simulink model "TST_CoTS_ThermDem"  (R2016b)
settings: Solver=FixedStepDiscrete  StartTime=0.0  StopTime=simTime  FixedStep=sampleTime  RelTol=1e-3
values from neighbouring files (symbols this model uses):
  testCase = 1    [initTST_CoTS_ThermDem_001.m]
libraries: simulink x4, UnitTest_Lib x2
settings Model: Creator=xinchangran  LastModifiedBy=xinchangran
settings DebuggingCC: SignalRangeChecking=error

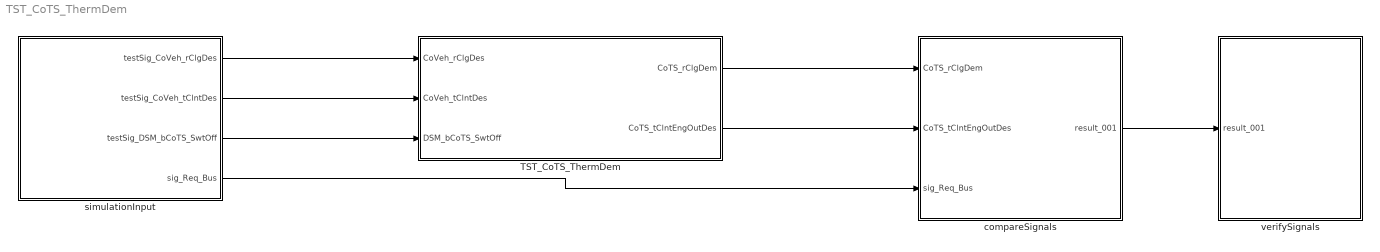
== system TST_CoTS_ThermDem ==
  TST_CoTS_ThermDem : Subsystem
  compareSignals : Subsystem
  simulationInput : Subsystem
  verifySignals : Subsystem
  wires:
  simulationInput/1(testSig_CoVeh_rClgDes) -> TST_CoTS_ThermDem/1(CoVeh_rClgDes)
  simulationInput/2(testSig_CoVeh_tClntDes) -> TST_CoTS_ThermDem/2(CoVeh_tClntDes)
  simulationInput/3(testSig_DSM_bCoTS_SwtOff) -> TST_CoTS_ThermDem/3(DSM_bCoTS_SwtOff)
  TST_CoTS_ThermDem/1(CoTS_rClgDem) -> compareSignals/1(CoTS_rClgDem)
  TST_CoTS_ThermDem/2(CoTS_tClntEngOutDes) -> compareSignals/2(CoTS_tClntEngOutDes)
  simulationInput/4(sig_Req_Bus) -> compareSignals/3(sig_Req_Bus)
  compareSignals/1(result_001) -> verifySignals/1(result_001)

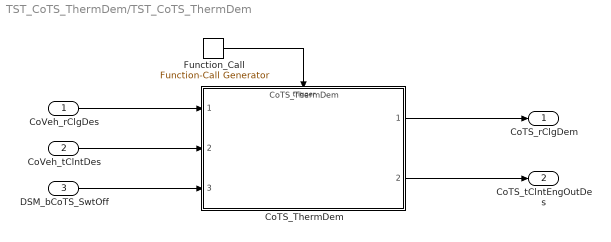
== system TST_CoTS_ThermDem/TST_CoTS_ThermDem ==
  CoVeh_rClgDes : Inport
  CoVeh_tClntDes : Inport  Port=2
  DSM_bCoTS_SwtOff : Inport  Port=3
  CoTS_ThermDem : ModelReference  ModelNameDialog=CoTS_ThermDem  SimulationMode=Normal  ModelReferenceVersion=1.28  TriggerPortName=function  TriggerPortTriggerType=function-call  TriggerPortStatesWhenEnabling=held
  Function_Call : simulink/Ports & Subsystems/Function-Call Generator  sample_time=sampleTime  numberOfIterations=1
  CoTS_rClgDem : Outport
  CoTS_tClntEngOutDes : Outport  Port=2
  wires:
  Function_Call/1 -> CoTS_ThermDem/Trigger
  CoVeh_rClgDes/1 -> CoTS_ThermDem/1
  CoVeh_tClntDes/1 -> CoTS_ThermDem/2
  DSM_bCoTS_SwtOff/1 -> CoTS_ThermDem/3
  CoTS_ThermDem/1 -> CoTS_rClgDem/1
  CoTS_ThermDem/2 -> CoTS_tClntEngOutDes/1

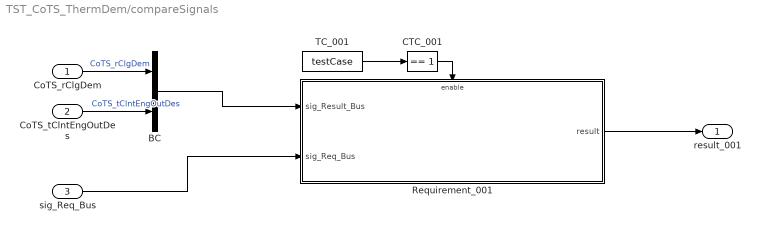
== system TST_CoTS_ThermDem/compareSignals ==
  CoTS_rClgDem : Inport
  CoTS_tClntEngOutDes : Inport  Port=2
  sig_Req_Bus : Inport  Port=3
  BC : BusCreator  Inputs=2
  CTC_001 : simulink/Logic and Bit Operations/Compare To Constant  relop===  const=1  OutDataTypeStr=boolean
  Requirement_001 : Subsystem
  TC_001 : Constant  Value=testCase
  result_001 : Outport
  wires:
  CoTS_rClgDem/1 -> BC/1  "CoTS_rClgDem"
  CoTS_tClntEngOutDes/1 -> BC/2  "CoTS_tClntEngOutDes"
  TC_001/1 -> CTC_001/1
  CTC_001/1 -> Requirement_001/Enable
  sig_Req_Bus/1 -> Requirement_001/2(sig_Req_Bus)
  BC/1 -> Requirement_001/1(sig_Result_Bus)
  Requirement_001/1(result) -> result_001/1

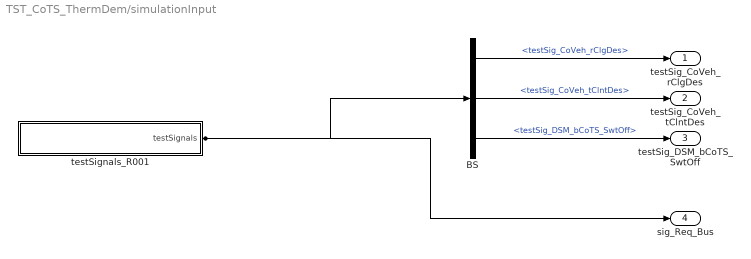
== system TST_CoTS_ThermDem/simulationInput ==
  BS : BusSelector  OutputSignals=testSig_CoVeh_rClgDes,testSig_CoVeh_tClntDes,testSig_DSM_bCoTS_SwtOff
  testSignals_R001 : Subsystem
  testSig_CoVeh_rClgDes : Outport
  testSig_CoVeh_tClntDes : Outport  Port=2
  testSig_DSM_bCoTS_SwtOff : Outport  Port=3
  sig_Req_Bus : Outport  Port=4
  wires:
  BS/1 -> testSig_CoVeh_rClgDes/1  "<testSig_CoVeh_rClgDes>"
  BS/2 -> testSig_CoVeh_tClntDes/1  "<testSig_CoVeh_tClntDes>"
  BS/3 -> testSig_DSM_bCoTS_SwtOff/1  "<testSig_DSM_bCoTS_SwtOff>"
  testSignals_R001/1(testSignals) -> BS/1, sig_Req_Bus/1

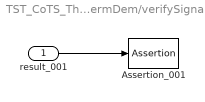
== system TST_CoTS_ThermDem/verifySignals ==
  result_001 : Inport
  Assertion_001 : Assertion  Enabled=off
  wires:
  result_001/1 -> Assertion_001/1

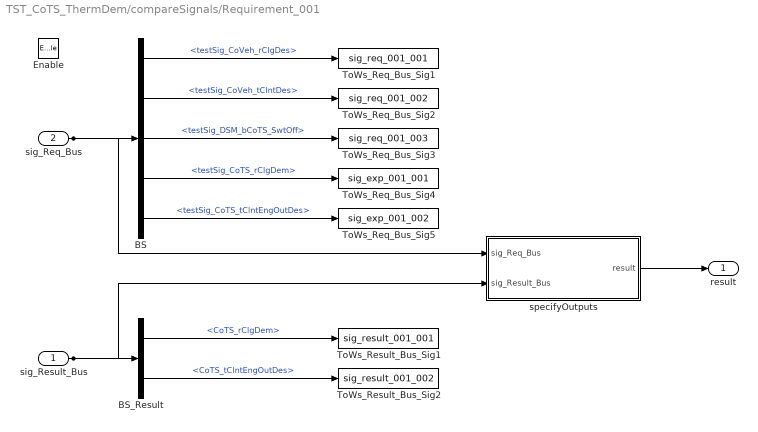
== system TST_CoTS_ThermDem/compareSignals/Requirement_001 ==
  sig_Result_Bus : Inport
  sig_Req_Bus : Inport  Port=2
  Enable : EnablePort
  BS : BusSelector  OutputSignals=testSig_CoVeh_rClgDes,testSig_CoVeh_tClntDes,testSig_DSM_bCoTS_SwtOff,testSig_CoTS_rClgDem,testSig_CoTS_tClntEngOutDes
  BS_Result : BusSelector  OutputSignals=CoTS_rClgDem,CoTS_tClntEngOutDes
  ToWs_Req_Bus_Sig1 : ToWorkspace  VariableName=sig_req_001_001  SaveFormat=Structure With Time
  ToWs_Req_Bus_Sig2 : ToWorkspace  VariableName=sig_req_001_002  SaveFormat=Structure With Time
  ToWs_Req_Bus_Sig3 : ToWorkspace  VariableName=sig_req_001_003  SaveFormat=Structure With Time
  ToWs_Req_Bus_Sig4 : ToWorkspace  VariableName=sig_exp_001_001  SaveFormat=Structure With Time
  ToWs_Req_Bus_Sig5 : ToWorkspace  VariableName=sig_exp_001_002  SaveFormat=Structure With Time
  ToWs_Result_Bus_Sig1 : ToWorkspace  VariableName=sig_result_001_001  SaveFormat=Structure With Time
  ToWs_Result_Bus_Sig2 : ToWorkspace  VariableName=sig_result_001_002  SaveFormat=Structure With Time
  specifyOutputs : Subsystem
  result : Outport
  wires:
  sig_Req_Bus/1 -> BS/1, specifyOutputs/1(sig_Req_Bus)
  BS/1 -> ToWs_Req_Bus_Sig1/1  "<testSig_CoVeh_rClgDes>"
  BS/2 -> ToWs_Req_Bus_Sig2/1  "<testSig_CoVeh_tClntDes>"
  BS/3 -> ToWs_Req_Bus_Sig3/1  "<testSig_DSM_bCoTS_SwtOff>"
  BS/4 -> ToWs_Req_Bus_Sig4/1  "<testSig_CoTS_rClgDem>"
  BS/5 -> ToWs_Req_Bus_Sig5/1  "<testSig_CoTS_tClntEngOutDes>"
  sig_Result_Bus/1 -> BS_Result/1, specifyOutputs/2(sig_Result_Bus)
  BS_Result/1 -> ToWs_Result_Bus_Sig1/1  "<CoTS_rClgDem>"
  BS_Result/2 -> ToWs_Result_Bus_Sig2/1  "<CoTS_tClntEngOutDes>"
  specifyOutputs/1(result) -> result/1

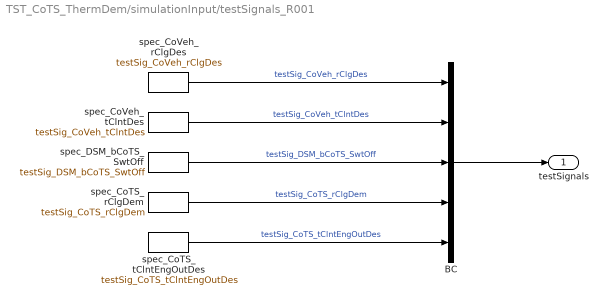
== system TST_CoTS_ThermDem/simulationInput/testSignals_R001 ==
  BC : BusCreator  Inputs=5
  spec_CoTS_rClgDem : FromWorkspace  VariableName=testSig_CoTS_rClgDem  Interpolate=off  OutputAfterFinalValue=Holding final value
  spec_CoTS_tClntEngOutDes : FromWorkspace  VariableName=testSig_CoTS_tClntEngOutDes  Interpolate=off  OutputAfterFinalValue=Holding final value
  spec_CoVeh_rClgDes : FromWorkspace  VariableName=testSig_CoVeh_rClgDes  Interpolate=off  OutputAfterFinalValue=Holding final value
  spec_CoVeh_tClntDes : FromWorkspace  VariableName=testSig_CoVeh_tClntDes  Interpolate=off  OutputAfterFinalValue=Holding final value
  spec_DSM_bCoTS_SwtOff : FromWorkspace  VariableName=testSig_DSM_bCoTS_SwtOff  Interpolate=off  OutputAfterFinalValue=Holding final value
  testSignals : Outport
  wires:
  BC/1 -> testSignals/1
  spec_CoVeh_rClgDes/1 -> BC/1  "testSig_CoVeh_rClgDes"
  spec_CoVeh_tClntDes/1 -> BC/2  "testSig_CoVeh_tClntDes"
  spec_DSM_bCoTS_SwtOff/1 -> BC/3  "testSig_DSM_bCoTS_SwtOff"
  spec_CoTS_rClgDem/1 -> BC/4  "testSig_CoTS_rClgDem"
  spec_CoTS_tClntEngOutDes/1 -> BC/5  "testSig_CoTS_tClntEngOutDes"

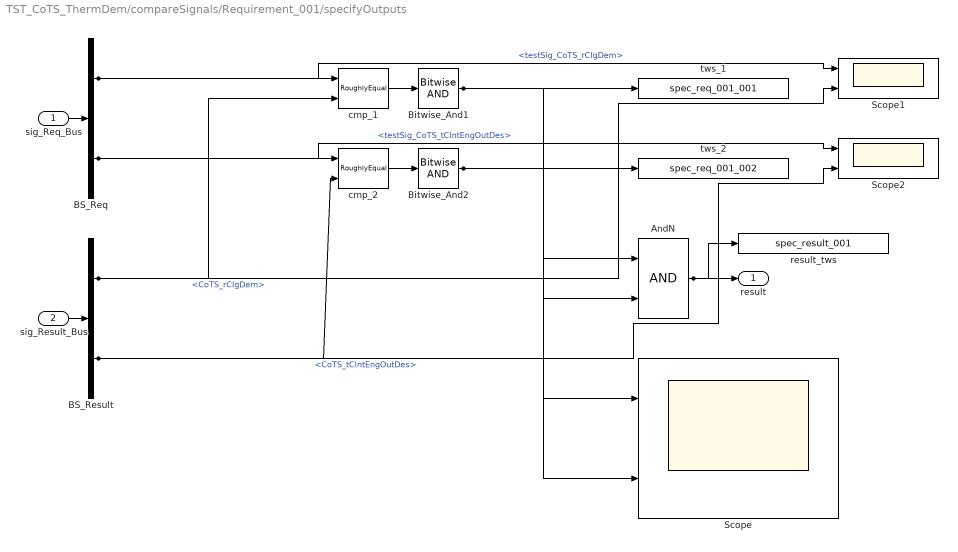
== system TST_CoTS_ThermDem/compareSignals/Requirement_001/specifyOutputs ==
  sig_Req_Bus : Inport
  sig_Result_Bus : Inport  Port=2
  AndN : Logic
  BS_Req : BusSelector  OutputSignals=testSig_CoTS_rClgDem,testSig_CoTS_tClntEngOutDes
  BS_Result : BusSelector  OutputSignals=CoTS_rClgDem,CoTS_tClntEngOutDes
  Bitwise_And1 : simulink/Logic and Bit Operations/Bitwise Operator  logicop=AND  UseBitMask=off  BitMask=bin2dec('11011001')  BitMaskRealWorld=Stored Integer
  Bitwise_And2 : simulink/Logic and Bit Operations/Bitwise Operator  logicop=AND  UseBitMask=off  BitMask=bin2dec('11011001')  BitMaskRealWorld=Stored Integer
  Scope : Scope  NumInputPorts=2
  Scope1 : Scope  NumInputPorts=2
  Scope2 : Scope  NumInputPorts=2
  cmp_1 : UnitTest_Lib/RoughlyEqual  slope=0.1
  cmp_2 : UnitTest_Lib/RoughlyEqual  slope=0.1
  result_tws : ToWorkspace  VariableName=spec_result_001
  tws_1 : ToWorkspace  VariableName=spec_req_001_001
  tws_2 : ToWorkspace  VariableName=spec_req_001_002
  result : Outport
  wires:
  sig_Req_Bus/1 -> BS_Req/1
  sig_Result_Bus/1 -> BS_Result/1
  AndN/1 -> result/1, result_tws/1
  BS_Req/1 -> cmp_1/1, Scope1/1  "<testSig_CoTS_rClgDem>"
  BS_Result/1 -> cmp_1/2, Scope1/2  "<CoTS_rClgDem>"
  cmp_1/1 -> Bitwise_And1/1
  Bitwise_And1/1 -> tws_1/1, AndN/1, Scope/1
  BS_Req/2 -> cmp_2/1, Scope2/1  "<testSig_CoTS_tClntEngOutDes>"
  BS_Result/2 -> cmp_2/2, Scope2/2  "<CoTS_tClntEngOutDes>"
  cmp_2/1 -> Bitwise_And2/1
  Bitwise_And2/1 -> tws_2/1, AndN/2, Scope/2
